simulink library "nmc"  (R2015b)
settings: Solver=ode45  SolverMode=SingleTasking  StartTime=0.0  StopTime=10.0  RelTol=1e-3
undefined symbols (not defined in the file): c, c_jointstop, CtrlPar_FP_List, CtrlPar_FP_R_List, CtrlPar_LL_List, CtrlPar_St_List, CtrlPar_St_R_List, CtrlPar_Sw_List, CtrlPar_Sw_R_List, CtrlPar_theta0_List, CtrlPar_Tr_List, CtrlPar_Tr_R_List, CtrlPar_VelocityFile_List, D1G_HAT, eref, FmaxBFSH, FmaxGAS, FmaxGLU, FmaxHAB, FmaxHAD, FmaxHAM, FmaxHFL, FmaxRF, FmaxSOL, FmaxTA, FmaxVAS, init_a_tgt, init_a_tgtR, K, leg_l, LongDelay, LongLoopDelay, loptBFSH, loptGAS, loptGLU, loptHAB, loptHAD, loptHAM, loptHFL, loptRF, loptSOL, loptTA, loptVAS, lslackBFSH, lslackGAS, lslackGLU, lslackHAB, lslackHAD, lslackHAM, lslackHFL, lslackRF, lslackSOL, lslackTA, lslackVAS, magnitude, maxLoad_control_List, MidDelay, N, phi12_LowLimit, phi12_UpLimit ... (+96)
libraries: nmc x63, simulink_extras x30, simulink x15, LopesDevelopmentLibrary x3
(part 2 of 10)

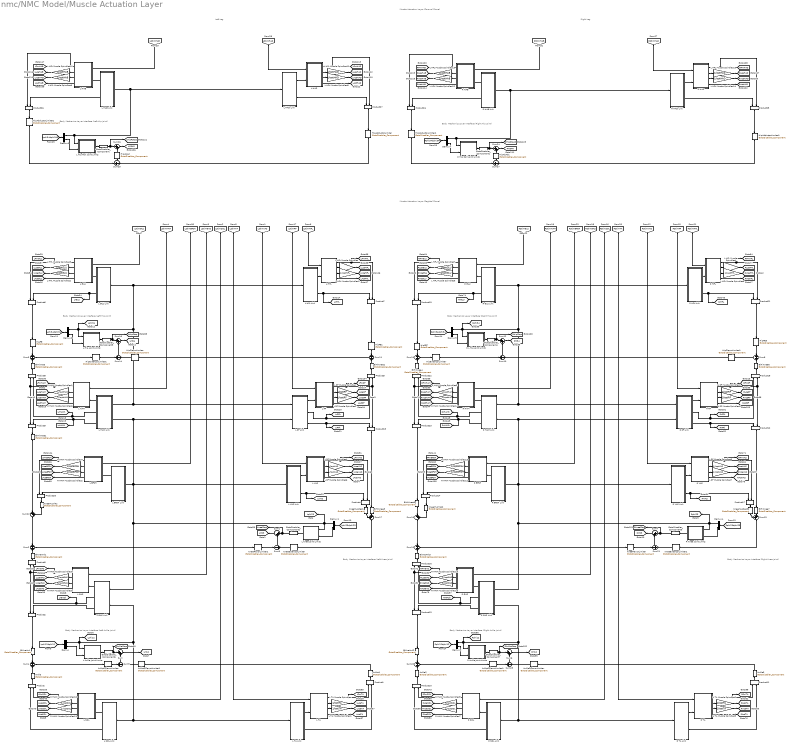
== system nmc/NMC Model/Muscle Actuation Layer ==
  note: Muscle Actuation Layer
      | (Sagittal Plane)
  note: Body Mechanics Layer
      | Interface (Left Hip Joint)
  note: Body Mechanics Layer
      | Interface (Left Knee Joint)
  note: Body Mechanics Layer
      | Interface (Left Ankle Joint)
  note: Body Mechanics Layer
      | Interface (Right Hip Joint)
  note: Body Mechanics Layer
      | Interface (Right Knee Joint)
  note: Body Mechanics Layer
      | Interface (Right Ankle Joint)
  note: Left Leg
  note: Body Mechanics Layer
      | Interface (Left Hip Joint)
  note: Body Mechanics Layer
      | Interface (Right Hip Joint)
  note: Right Leg
  note: Muscle Actuation Layer
      | (Coronal Plane)
  Ankle{,1..3} (4 alike) : nmc/GotoDisabler_Component  GotoTag=NMC_AnkleMuscles_Percentage
  AnkleDFlexorLimiter : nmc/GotoDisabler_Component  GotoTag=NMC_AnkleDFlexor_Percentage
  AnkleDFlexorLimiter1 : nmc/GotoDisabler_Component  GotoTag=NMC_AnkleDFlexor_Percentage
  AnklePFlexorLimiter : nmc/GotoDisabler_Component  GotoTag=NMC_AnklePFlexor_Percentage
  AnklePFlexorLimiter1 : nmc/GotoDisabler_Component  GotoTag=NMC_AnklePFlexor_Percentage
  BiHiKnee{,1..7} (8 alike) : nmc/GotoDisabler_Component  GotoTag=NMC_BiArticularMuscles_HK_Percentage
  BiKneAnk{,1..3} (4 alike) : nmc/GotoDisabler_Component  GotoTag=NMC_BiArticularMuscles_KA_Percentage
  Demux{,1..7} (8 alike) : Demux  Outputs=2
  GotoDisabler_Component{,1..7} (8 alike) : nmc/GotoDisabler_Component  GotoTag=DisableNMC_JointLimits
  HipAbAd : nmc/GotoDisabler_Component  GotoTag=NMC_HipAbAdMuscles_Percentage
  HipAbAd1 : nmc/GotoDisabler_Component  GotoTag=NMC_HipAbAdMuscles_Percentage
  HipAbductorLimiter1 : nmc/GotoDisabler_Component  GotoTag=NMC_HipAbductor_Percentage
  HipAbductorLimiter2 : nmc/GotoDisabler_Component  GotoTag=NMC_HipAbductor_Percentage
  HipAdductorLimiter : nmc/GotoDisabler_Component  GotoTag=NMC_HipAdductor_Percentage
  HipAdductorLimiter1 : nmc/GotoDisabler_Component  GotoTag=NMC_HipAdductor_Percentage
  HipExtensorLimiter : nmc/GotoDisabler_Component  GotoTag=NMC_HipExtensor_Percentage
  HipExtensorLimiter1 : nmc/GotoDisabler_Component  GotoTag=NMC_HipExtensor_Percentage
  HipFE{,1..3} (4 alike) : nmc/GotoDisabler_Component  GotoTag=NMC_HipFEMuscles_Percentage
  HipFlexorLimiter : nmc/GotoDisabler_Component  GotoTag=NMC_HipFlexor_Percentage
  HipFlexorLimiter1 : nmc/GotoDisabler_Component  GotoTag=NMC_HipFlexor_Percentage
  KneeExtensorLimiter : nmc/GotoDisabler_Component  GotoTag=NMC_KneeExtensor_Percentage
  KneeExtensorLimiter1 : nmc/GotoDisabler_Component  GotoTag=NMC_KneeExtensor_Percentage
  KneeFlexorLimiter : nmc/GotoDisabler_Component  GotoTag=NMC_KneeFlexor_Percentage
  KneeFlexorLimiter1 : nmc/GotoDisabler_Component  GotoTag=NMC_KneeFlexor_Percentage
  KneeMuscles{,1..3} (4 alike) : nmc/GotoDisabler_Component  GotoTag=NMC_KneeMuscles_Percentage
  L Ankle Joint Limits : Subsystem
  L BFSH : Subsystem
  L BFSH Link : Subsystem
  L GAS : Subsystem
  L GAS Link : Subsystem
  L GLU : Subsystem
  L GLU Link : Subsystem
  L HAB : Subsystem
  L HAB Link : Subsystem
  L HAD : Subsystem
  L HAD Link : Subsystem
  L HAM : Subsystem
  L HAM Link : Subsystem
  L HFL : Subsystem
  L HFL Muscle Spindles{,1,4..5} (4 alike) : Gain  Gain=1/loptHFL
  L HFL Muscle Spindles{9..10,12..13} (4 alike) : Gain  Gain=1/loptHAB
  L HFL Muscle Spindles{8,11,14..15} (4 alike) : Gain  Gain=1/loptHAD
  L HFL Muscle Spindles{2..3,6..7} (4 alike) : Gain  Gain=1/loptGLU
  L HFL Link : Subsystem
  L Hip Joint Limits : Subsystem
  L Hip Roll Joint Limits : Subsystem
  L Knee Joint Limits : Subsystem
  L RF : Subsystem
  L RF Muscle Spindles{,1..3} (4 alike) : Gain  Gain=1/loptRF
  L RF Muscle Spindles{4..7} (4 alike) : Gain  Gain=1/loptVAS
  L RF Link : Subsystem
  L SOL : Subsystem
  L SOL Link : Subsystem
  L TA : Subsystem
  L TA Muscle Spindles{,1..3} (4 alike) : Gain  Gain=1/loptTA
  L TA Link : Subsystem
  L VAS : Subsystem
  L VAS Link : Subsystem
  Product{,1..27} (28 alike) : Product  RndMeth=Zero
  R Ankle Joint Limits : Subsystem
  R BFSH : Subsystem
  R BFSH Link : Subsystem
  R GAS : Subsystem
  R GAS Link : Subsystem
  R GLU : Subsystem
  R GLU Link : Subsystem
  R HAB : Subsystem
  R HAB Link : Subsystem
  R HAD : Subsystem
  R HAD Link : Subsystem
  R HAM : Subsystem
  R HAM Muscle Spindles{1,3,6,14} (4 alike) : Gain  Gain=1/loptHAM
  R HAM Muscle Spindles{5,7,10..11} (4 alike) : Gain  Gain=1/loptSOL
  R HAM Muscle Spindles{2,4,12..13} (4 alike) : Gain  Gain=1/loptBFSH
  R HAM Muscle Spindles{8..9,15..16} (4 alike) : Gain  Gain=1/loptGAS
  R HAM Link : Subsystem
  R HFL : Subsystem
  R HFL Link : Subsystem
  R Hip Roll Joint Limits : Subsystem
  R Knee Joint Limits : Subsystem
  R L Hip Joint Limits : Subsystem
  R RF : Subsystem
  R RF Link : Subsystem
  R SOL : Subsystem
  R SOL Link : Subsystem
  R TA : Subsystem
  R TA Link : Subsystem
  R VAS : Subsystem
  R VAS Link : Subsystem
  Sum{,1,6..7,12,16,18,22,24,26} (10 alike) : Sum  Inputs=|++
  Sum{9..10,14,23,25,27} (6 alike) : Sum  Inputs=+-
  Sum{2..4,8,11,15,19..20} (8 alike) : Sum
  Sum13 : Sum  Inputs=++|
  Sum17 : Sum  Inputs=++|
  Sum21 : Sum  Inputs=-+
  Sum5 : Sum  Inputs=-+
  tag scope: LActBFSH=global, LActGAS=global, LActGLU=global, LActHAB=global, LActHAD=global, LActHAM=global, LActHFL=global, LActRF=global, LActSOL=global, LActTA=global, LActVAS=global, LAnkleStop=global, LFmBFSH=global, LFmGAS=global, LFmGLU=global, LFmHAB=global, LFmHAD=global, LFmHAM=global, LFmHFL=global, LFmRF=global, LFmSOL=global, LFmTA=global, LFmVAS=global, LHipRStop=global, LHipStop=global, LKneeStop=global, LLceBFSH=global, LLceGAS=global, LLceGLU=global, LLceHAB=global, LLceHAD=global, LLceHAM=global, LLceHFL=global, LLceRF=global, LLceSOL=global, LLceTA=global, LLceVAS=global, LM12=global, LM23=global, LM34=global, LM34R=global, LVceBFSH=global, LVceGAS=global, LVceGLU=global, LVceHAB=global, LVceHAD=global, LVceHAM=global, LVceHFL=global, LVceRF=global, LVceSOL=global, LVceTA=global, LVceVAS=global, Lphi12=global, Lphi23=global, Lphi34=global, LrGASk=global, LrGLU=global, LrHAMh=global, LrHAMk=global, LrHFL=global, LrRFh=global, LrRFk=global, LrVAS=global, RActBFSH=global, RActGAS=global, RActGLU=global, RActHAB=global, RActHAD=global, RActHAM=global, RActHFL=global, RActRF=global, RActSOL=global, RActTA=global, RActVAS=global, RAnkleStop=global, RFmBFSH=global, RFmGAS=global, RFmGLU=global, RFmHAB=global, RFmHAD=global, RFmHAM=global, RFmHFL=global, RFmRF=global, RFmSOL=global, RFmTA=global, RFmVAS=global, RHipStop=global, RHipStopR=global, RKneeStop=global, RLceBFSH=global, RLceGAS=global, RLceGLU=global, RLceHAB=global, RLceHAD=global, RLceHAM=global, RLceHFL=global, RLceRF=global, RLceSOL=global, RLceTA=global, RLceVAS=global, RM12=global, RM23=global, RM34=global, RM34R=global, RVceBFSH=global, RVceGAS=global, RVceGLU=global, RVceHAB=global, RVceHAD=global, RVceHAM=global, RVceHFL=global, RVceRF=global, RVceSOL=global, RVceTA=global, RVceVAS=global, Rphi12=global, Rphi23=global, Rphi34=global, RrGASk=global, RrGLU=global, RrHAMh=global, RrHAMk=global, RrHFL=global, RrRFh=global, RrRFk=global, RrVAS=global
  wires:
  Demux1/1 -> L Knee Joint Limits/1(phi [rad]), L VAS Link/1(phi23 [rad]), L RF Link/2(phi23 [rad]), L HAM Link/2(phi23 [rad]), L BFSH Link/1(phi23 [rad]), L GAS Link/1(phi23 [rad]), [Lphi23]
  L SOL/1(Fmtc) -> Product/2, [LFmSOL]
  L TA/2(Lce) -> L TA Muscle Spindles/1
  L TA/4(A) -> [LActTA]
  L GAS/1(Fmtc) -> Product2/1, Product3/1, [LFmGAS]
  Demux/1 -> L SOL Link/1(phi12 [rad]), L TA Link/1(phi12 [rad]), L GAS Link/2(phi12 [rad]), L Ankle Joint Limits/1(phi [rad]), [Lphi12]
  [LStimTA] -> L TA/1(STIM)
  [LStimSOL] -> L SOL/1(STIM)
  [LStimHAM] -> L HAM/1(STIM)
  L HAM/1(Fmtc) -> Product9/1, Product8/1, [LFmHAM]
  L HAM/2(Lce) -> R HAM Muscle Spindles1/1
  L HFL/2(Lce) -> L HFL Muscle Spindles/1
  L GLU/1(Fmtc) -> Product6/1, [LFmGLU]
  [LStimGLU] -> L GLU/1(STIM)
  Sum16/1 -> [LM34]
  Demux/2 -> L Ankle Joint Limits/2(dphi [rad/s])
  Sum9/1 -> Sum/2
  Demux1/2 -> L Knee Joint Limits/2(dphi [rad/s])
  L SOL Link/1(lmtc [m]) -> L SOL/2(lmtc [m])
  L TA Link/1(lmtc [m]) -> L TA/2(lmtc [m])
  L GAS Link/3(lever12 [m]) -> Product2/2
  L GAS Link/2(lever23 [m]) -> Product3/2, [LrGASk]
  [LStimGAS] -> L GAS/1(STIM)
  L GAS Link/1(lmtu [m]) -> L GAS/2(lmtc [m])
  L VAS Link/1(lmtu [m]) -> L VAS/2(lmtc [m])
  L HAM Link/1(lmtu [m]) -> L HAM/2(lmtc [m])
  L HAM Link/2(lever34 [m]) -> Product8/2, [LrHAMh]
  L HAM Link/3(lever23 [m]) -> Product9/2, [LrHAMk]
  Sum3/1 -> HipExtensorLimiter1/1
  Sum4/1 -> AnklePFlexorLimiter/1
  [Lphi12dphi12] -> Demux/1
  [Lphi23dphi23] -> Demux1/1
  [Lphi34dphi34] -> Demux2/1
  Demux2/1 -> L Hip Joint Limits/1(phi [rad]), L HFL Link/1(phi34 [rad]), L GLU Link/1(phi34 [rad]), L RF Link/1(phi34 [rad]), L HAM Link/1(phi34 [rad]), [Lphi34]
  L SOL Link/2(lever [m]) -> Product/1
  Product2/1 -> BiKneAnk/1
  L TA Link/2(lever [m]) -> Product1/2
  L Ankle Joint Limits/1(M_stop [Nm]) -> GotoDisabler_Component6/1
  L SOL/4(A) -> [LActSOL]
  L GAS/4(A) -> [LActGAS]
  L VAS/4(A) -> [LActVAS]
  L VAS/1(Fmtc) -> Product4/2, [LFmVAS]
  Sum1/1 -> [LM23]
  L Knee Joint Limits/1(M_stop [Nm]) -> GotoDisabler_Component2/1
  Sum5/1 -> Sum1/2
  L VAS Link/2(lever [m]) -> [LrVAS], Product4/1
  Sum2/1 -> KneeFlexorLimiter1/1
  L HAM/4(A) -> [LActHAM]
  L GLU Link/1(lmtu [m]) -> L GLU/2(lmtc [m])
  L GLU Link/2(lever [m]) -> Product6/2, [LrGLU]
  L GLU/4(A) -> [LActGLU]
  Demux2/2 -> L Hip Joint Limits/2(dphi [rad/s])
  Sum14/1 -> Sum16/2
  L HFL Link/1(lmtu [m]) -> L HFL/2(lmtc [m])
  L HFL/4(A) -> [LActHFL]
  L HFL Link/2(lever [m]) -> Product7/1, [LrHFL]
  [LStimVAS] -> L VAS/1(STIM)
  L GLU/2(Lce) -> L HFL Muscle Spindles3/1
  L GLU/3(Vce) -> L HFL Muscle Spindles2/1
  L HAM/3(Vce) -> R HAM Muscle Spindles6/1
  L GAS/3(Vce) -> R HAM Muscle Spindles9/1
  L GAS/2(Lce) -> R HAM Muscle Spindles8/1
  L SOL/2(Lce) -> R HAM Muscle Spindles10/1
  L SOL/3(Vce) -> R HAM Muscle Spindles11/1
  L TA/3(Vce) -> L TA Muscle Spindles1/1
  L VAS/3(Vce) -> L RF Muscle Spindles6/1
  L VAS/2(Lce) -> L RF Muscle Spindles4/1
  L HFL/3(Vce) -> L HFL Muscle Spindles1/1
  L RF/4(A) -> [LActRF]
  L RF/3(Vce) -> L RF Muscle Spindles2/1
  L RF/2(Lce) -> L RF Muscle Spindles/1
  L RF Link/1(lmtu [m]) -> L RF/2(lmtc [m])
  L RF Link/2(lever34 [m]) -> Product5/1, [LrRFh]
  L RF Link/3(lever23 [m]) -> Product15/1, [LrRFk]
  [LStimRF] -> L RF/1(STIM)
  Product5/1 -> BiHiKnee2/1
  Product15/1 -> BiHiKnee3/1
  Sum17/1 -> KneeExtensorLimiter/1
  [LStimBFSH] -> L BFSH/1(STIM)
  L BFSH Link/1(lmtu [m]) -> L BFSH/2(lmtc [m])
  L BFSH Link/2(lever [m]) -> Product20/2
  L BFSH/4(A) -> [LActBFSH]
  L BFSH/2(Lce) -> R HAM Muscle Spindles4/1
  L BFSH/3(Vce) -> R HAM Muscle Spindles2/1
  L HFL Muscle Spindles1/1 -> [LVceHFL]
  L HFL Muscle Spindles2/1 -> [LVceGLU]
  L HFL Muscle Spindles3/1 -> [LLceGLU]
  L RF Muscle Spindles6/1 -> [LVceVAS]
  L RF/1(Fmtc) -> Product5/2, Product15/2, [LFmRF]
  L BFSH/1(Fmtc) -> Product20/1, [LFmBFSH]
  R HAM Muscle Spindles8/1 -> [LLceGAS]
  R HAM Muscle Spindles9/1 -> [LVceGAS]
  R HAM Muscle Spindles10/1 -> [LLceSOL]
  R HAM Muscle Spindles11/1 -> [LVceSOL]
  L TA/1(Fmtc) -> Product1/1, [LFmTA]
  L TA Muscle Spindles1/1 -> [LVceTA]
  L HFL Muscle Spindles/1 -> [LLceHFL]
  R HAM Muscle Spindles1/1 -> [LLceHAM]
  R HAM Muscle Spindles6/1 -> [LVceHAM]
  L RF Muscle Spindles/1 -> [LLceRF]
  L RF Muscle Spindles2/1 -> [LVceRF]
  R HAM Muscle Spindles4/1 -> [LLceBFSH]
  R HAM Muscle Spindles2/1 -> [LVceBFSH]
  L RF Muscle Spindles4/1 -> [LLceVAS]
  L TA Muscle Spindles/1 -> [LLceTA]
  Demux4/1 -> R Knee Joint Limits/1(phi [rad]), R VAS Link/1(phi23 [rad]), R RF Link/2(phi23 [rad]), R HAM Link/2(phi23 [rad]), R BFSH Link/1(phi23 [rad]), R GAS Link/1(phi23 [rad]), [Rphi23]
  R SOL/1(Fmtc) -> Product10/2, [RFmSOL]
  R TA/2(Lce) -> L TA Muscle Spindles2/1
  R TA/4(A) -> [RActTA]
  R GAS/1(Fmtc) -> Product13/1, Product16/1, [RFmGAS]
  Demux3/1 -> R SOL Link/1(phi12 [rad]), R TA Link/1(phi12 [rad]), R GAS Link/2(phi12 [rad]), R Ankle Joint Limits/1(phi [rad]), [Rphi12]
  [RStimTA] -> R TA/1(STIM)
  [RStimSOL] -> R SOL/1(STIM)
  [RStimHAM] -> R HAM/1(STIM)
  R HAM/1(Fmtc) -> Product23/1, Product22/1, [RFmHAM]
  R HAM/2(Lce) -> R HAM Muscle Spindles3/1
  R HFL/1(Fmtc) -> Product21/2, [RFmHFL]
  R HFL/2(Lce) -> L HFL Muscle Spindles4/1
  [RStimHFL] -> R HFL/1(STIM)
  R GLU/1(Fmtc) -> Product19/1, [RFmGLU]
  [RStimGLU] -> R GLU/1(STIM)
  Sum12/1 -> [RM34]
  Demux3/2 -> R Ankle Joint Limits/2(dphi [rad/s])
  Sum23/1 -> Sum6/2
  Demux4/2 -> R Knee Joint Limits/2(dphi [rad/s])
  R SOL Link/1(lmtc [m]) -> R SOL/2(lmtc [m])
  R TA Link/1(lmtc [m]) -> R TA/2(lmtc [m])
  R GAS Link/3(lever12 [m]) -> Product13/2
  R GAS Link/2(lever23 [m]) -> Product16/2, [RrGASk]
  [RStimGAS] -> R GAS/1(STIM)
  R GAS Link/1(lmtu [m]) -> R GAS/2(lmtc [m])
  R VAS Link/1(lmtu [m]) -> R VAS/2(lmtc [m])
  R HAM Link/1(lmtu [m]) -> R HAM/2(lmtc [m])
  R HAM Link/2(lever34 [m]) -> Product22/2, [RrHAMh]
  R HAM Link/3(lever23 [m]) -> Product23/2, [RrHAMk]
  Sum19/1 -> HipExtensorLimiter/1
  Sum20/1 -> AnklePFlexorLimiter1/1
  [Rphi12dphi12] -> Demux3/1
  [Rphi23dphi23] -> Demux4/1
  [Rphi34dphi34] -> Demux5/1
  Demux5/1 -> R L Hip Joint Limits/1(phi [rad]), R HFL Link/1(phi34 [rad]), R GLU Link/1(phi34 [rad]), R RF Link/1(phi34 [rad]), R HAM Link/1(phi34 [rad]), [Rphi34]
  R SOL Link/2(lever [m]) -> Product10/1
  Product13/1 -> BiKneAnk2/1
  R TA Link/2(lever [m]) -> Product11/2
  Sum6/1 -> [RM12]
  R SOL/4(A) -> [RActSOL]
  R GAS/4(A) -> [RActGAS]
  R VAS/4(A) -> [RActVAS]
  R VAS/1(Fmtc) -> Product17/2, [RFmVAS]
  Sum7/1 -> [RM23]
  R Knee Joint Limits/1(M_stop [Nm]) -> GotoDisabler_Component3/1
  Sum21/1 -> Sum7/2
  R VAS Link/2(lever [m]) -> [RrVAS], Product17/1
  Sum15/1 -> KneeFlexorLimiter/1
  R HAM/4(A) -> [RActHAM]
  Product22/1 -> BiHiKnee4/1
  R GLU Link/1(lmtu [m]) -> R GLU/2(lmtc [m])
  R GLU Link/2(lever [m]) -> Product19/2, [RrGLU]
  R GLU/4(A) -> [RActGLU]
  Demux5/2 -> R L Hip Joint Limits/2(dphi [rad/s])
  Sum10/1 -> Sum12/2
  R HFL Link/1(lmtu [m]) -> R HFL/2(lmtc [m])
  R HFL/4(A) -> [RActHFL]
  R HFL Link/2(lever [m]) -> Product21/1, [RrHFL]
  [RStimVAS] -> R VAS/1(STIM)
  R GLU/2(Lce) -> L HFL Muscle Spindles7/1
  R GLU/3(Vce) -> L HFL Muscle Spindles6/1
  R HAM/3(Vce) -> R HAM Muscle Spindles14/1
  R GAS/3(Vce) -> R HAM Muscle Spindles16/1
  R GAS/2(Lce) -> R HAM Muscle Spindles15/1
  R SOL/2(Lce) -> R HAM Muscle Spindles5/1
  R SOL/3(Vce) -> R HAM Muscle Spindles7/1
  R TA/3(Vce) -> L TA Muscle Spindles3/1
  R VAS/3(Vce) -> L RF Muscle Spindles7/1
  R VAS/2(Lce) -> L RF Muscle Spindles5/1
  R HFL/3(Vce) -> L HFL Muscle Spindles5/1
  R RF/4(A) -> [RActRF]
  R RF/3(Vce) -> L RF Muscle Spindles3/1
  R RF/2(Lce) -> L RF Muscle Spindles1/1
  R RF Link/1(lmtu [m]) -> R RF/2(lmtc [m])
  R RF Link/2(lever34 [m]) -> Product18/1, [RrRFh]
  R RF Link/3(lever23 [m]) -> Product12/1, [RrRFk]
  [RStimRF] -> R RF/1(STIM)
  Sum8/1 -> HipFlexorLimiter1/1
  Product18/1 -> BiHiKnee6/1
  Product12/1 -> BiHiKnee7/1
  Sum13/1 -> KneeExtensorLimiter1/1
  [RStimBFSH] -> R BFSH/1(STIM)
  R BFSH Link/1(lmtu [m]) -> R BFSH/2(lmtc [m])
  R BFSH Link/2(lever [m]) -> Product14/2
  R BFSH/4(A) -> [RActBFSH]
  R BFSH/2(Lce) -> R HAM Muscle Spindles13/1
  R BFSH/3(Vce) -> R HAM Muscle Spindles12/1
  Sum18/1 -> Sum15/1
  Product23/1 -> BiHiKnee5/1
  L HFL Muscle Spindles5/1 -> [RVceHFL]
  L HFL Muscle Spindles6/1 -> [RVceGLU]
  L HFL Muscle Spindles7/1 -> [RLceGLU]
  L RF Muscle Spindles7/1 -> [RVceVAS]
  R RF/1(Fmtc) -> Product18/2, Product12/2, [RFmRF]
  R BFSH/1(Fmtc) -> Product14/1, [RFmBFSH]
  R HAM Muscle Spindles15/1 -> [RLceGAS]
  R HAM Muscle Spindles16/1 -> [RVceGAS]
  R HAM Muscle Spindles5/1 -> [RLceSOL]
  R HAM Muscle Spindles7/1 -> [RVceSOL]
  R TA/1(Fmtc) -> Product11/1, [RFmTA]
  L TA Muscle Spindles3/1 -> [RVceTA]
  L HFL Muscle Spindles4/1 -> [RLceHFL]
  R HAM Muscle Spindles3/1 -> [RLceHAM]
  R HAM Muscle Spindles14/1 -> [RVceHAM]
  L RF Muscle Spindles1/1 -> [RLceRF]
  L RF Muscle Spindles3/1 -> [RVceRF]
  R HAM Muscle Spindles13/1 -> [RLceBFSH]
  R HAM Muscle Spindles12/1 -> [RVceBFSH]
  L RF Muscle Spindles5/1 -> [RLceVAS]
  L TA Muscle Spindles2/1 -> [RLceTA]
  Sum11/1 -> HipFlexorLimiter/1
  [LStimHAD] -> L HAD/1(STIM)
  [LStimHAB] -> L HAB/1(STIM)
  Sum26/1 -> [LM34R]
  [Lphi34dphi34R] -> Demux6/1
  Demux6/1 -> L HAB Link/1(phi34R [rad]), L HAD Link/1(phi34R [rad]), L Hip Roll Joint Limits/1(phi [rad])
  Product26/1 -> HipAbductorLimiter2/1
  L HAB Link/1(lmtu [m]) -> L HAB/2(lmtc [m])
  L HAB Link/2(lever [m]) -> Product26/2
  Demux6/2 -> L Hip Roll Joint Limits/2(dphi [rad/s])
  L Hip Roll Joint Limits/1(M_stop [Nm]) -> GotoDisabler_Component/1
  Product27/1 -> HipAdductorLimiter/1
  L HAD Link/1(lmtu [m]) -> L HAD/2(lmtc [m])
  L HAD Link/2(lever [m]) -> Product27/1
  [RStimHAD] -> R HAD/1(STIM)
  Sum24/1 -> [RM34R]
  [Rphi34dphi34R] -> Demux7/1
  Demux7/1 -> R HAD Link/1(phi34R [rad]), R HAB Link/1(phi34R [rad]), R Hip Roll Joint Limits/1(phi [rad])
  Product24/1 -> HipAbductorLimiter1/1
  R HAB Link/1(lmtu [m]) -> R HAB/2(lmtc [m])
  R HAB Link/2(lever [m]) -> Product24/2
  Demux7/2 -> R Hip Roll Joint Limits/2(dphi [rad/s])
  R Hip Roll Joint Limits/1(M_stop [Nm]) -> GotoDisabler_Component1/1
  Product25/1 -> HipAdductorLimiter1/1
  R HAD Link/1(lmtu [m]) -> R HAD/2(lmtc [m])
  R HAD Link/2(lever [m]) -> Product25/1
  [RStimHAB] -> R HAB/1(STIM)
  L HAB/4(A) -> [LActHAB]
  L HAB/2(Lce) -> L HFL Muscle Spindles10/1
  L HAB/3(Vce) -> L HFL Muscle Spindles9/1
  L HFL Muscle Spindles9/1 -> [LVceHAB]
  L HFL Muscle Spindles10/1 -> [LLceHAB]
  L HAB/1(Fmtc) -> Product26/1, [LFmHAB]
  L HFL Muscle Spindles8/1 -> [LVceHAD]
  L HFL Muscle Spindles11/1 -> [LLceHAD]
  L HAD/2(Lce) -> L HFL Muscle Spindles11/1
  L HAD/3(Vce) -> L HFL Muscle Spindles8/1
  L HAD/4(A) -> [LActHAD]
  L HAD/1(Fmtc) -> [LFmHAD], Product27/2
  R HAB/4(A) -> [RActHAB]
  R HAB/2(Lce) -> L HFL Muscle Spindles13/1
  R HAB/3(Vce) -> L HFL Muscle Spindles12/1
  L HFL Muscle Spindles12/1 -> [RVceHAB]
  L HFL Muscle Spindles13/1 -> [RLceHAB]
  R HAB/1(Fmtc) -> [RFmHAB], Product24/1
  L HFL Muscle Spindles14/1 -> [RVceHAD]
  L HFL Muscle Spindles15/1 -> [RLceHAD]
  R HAD/2(Lce) -> L HFL Muscle Spindles15/1
  R HAD/3(Vce) -> L HFL Muscle Spindles14/1
  R HAD/4(A) -> [RActHAD]
  R HAD/1(Fmtc) -> [RFmHAD], Product25/2
  Sum/1 -> [LM12]
  GotoDisabler_Component7/1 -> Sum6/1, [RAnkleStop]
  GotoDisabler_Component6/1 -> Sum/1, [LAnkleStop]
  GotoDisabler_Component3/1 -> Sum7/1, [RKneeStop]
  GotoDisabler_Component2/1 -> Sum1/1, [LKneeStop]
  GotoDisabler_Component/1 -> Sum26/1, [LHipRStop]
  GotoDisabler_Component1/1 -> Sum24/1, [RHipStopR]
  R L Hip Joint Limits/1(M_stop [Nm]) -> GotoDisabler_Component4/1
  GotoDisabler_Component4/1 -> [RHipStop], Sum12/1
  L Hip Joint Limits/1(M_stop [Nm]) -> GotoDisabler_Component5/1
  GotoDisabler_Component5/1 -> Sum16/1, [LHipStop]
  R Ankle Joint Limits/1(M_stop [Nm]) -> GotoDisabler_Component7/1
  Product4/1 -> KneeMuscles1/1
  Product17/1 -> KneeMuscles3/1
  Product14/1 -> KneeMuscles2/1
  Product20/1 -> KneeMuscles/1
  Product21/1 -> HipFE3/1
  Product19/1 -> HipFE2/1
  Product6/1 -> HipFE/1
  Product/1 -> Ankle/1
  Product10/1 -> Ankle2/1
  Product11/1 -> Ankle3/1
  Product1/1 -> Ankle1/1
  HipAbductorLimiter2/1 -> Sum25/1
  HipAbductorLimiter1/1 -> Sum27/1
  HipAdductorLimiter/1 -> Sum25/2
  HipAdductorLimiter1/1 -> Sum27/2
  Product9/1 -> BiHiKnee1/1
  KneeFlexorLimiter1/1 -> Sum5/1
  KneeExtensorLimiter/1 -> Sum5/2
  KneeFlexorLimiter/1 -> Sum21/1
  KneeExtensorLimiter1/1 -> Sum21/2
  AnklePFlexorLimiter1/1 -> Sum23/1
  AnklePFlexorLimiter/1 -> Sum9/1
  HipExtensorLimiter1/1 -> Sum14/1
  HipFlexorLimiter/1 -> Sum14/2
  HipExtensorLimiter/1 -> Sum10/1
  HipFlexorLimiter1/1 -> Sum10/2
  AnkleDFlexorLimiter1/1 -> Sum9/2
  AnkleDFlexorLimiter/1 -> Sum23/2
  Sum25/1 -> HipAbAd/1
  HipAbAd/1 -> Sum26/2
  Sum27/1 -> HipAbAd1/1
  HipAbAd1/1 -> Sum24/2
  HipFE/1 -> Sum3/1
  HipFE1/1 -> Sum11/1
  HipFE2/1 -> Sum19/1
  HipFE3/1 -> Sum8/1
  BiHiKnee/1 -> Sum3/2
  Product8/1 -> BiHiKnee/1
  BiHiKnee1/1 -> Sum22/1
  BiHiKnee2/1 -> Sum11/2
  BiHiKnee3/1 -> Sum17/2
  BiHiKnee4/1 -> Sum19/2
  BiHiKnee5/1 -> Sum18/1
  BiHiKnee6/1 -> Sum8/2
  BiHiKnee7/1 -> Sum13/2
  Sum22/1 -> Sum2/1
  KneeMuscles/1 -> Sum22/2
  KneeMuscles1/1 -> Sum17/1
  KneeMuscles2/1 -> Sum18/2
  KneeMuscles3/1 -> Sum13/1
  BiKneAnk/1 -> Sum4/1
  Product3/1 -> BiKneAnk1/1
  BiKneAnk1/1 -> Sum2/2
  BiKneAnk2/1 -> Sum20/1
  Product16/1 -> BiKneAnk3/1
  BiKneAnk3/1 -> Sum15/2
  Ankle/1 -> Sum4/2
  Ankle1/1 -> AnkleDFlexorLimiter1/1
  Ankle2/1 -> Sum20/2
  Ankle3/1 -> AnkleDFlexorLimiter/1
  Product7/1 -> HipFE1/1
  [LStimHFL] -> L HFL/1(STIM)
  L HFL/1(Fmtc) -> Product7/2, [LFmHFL]

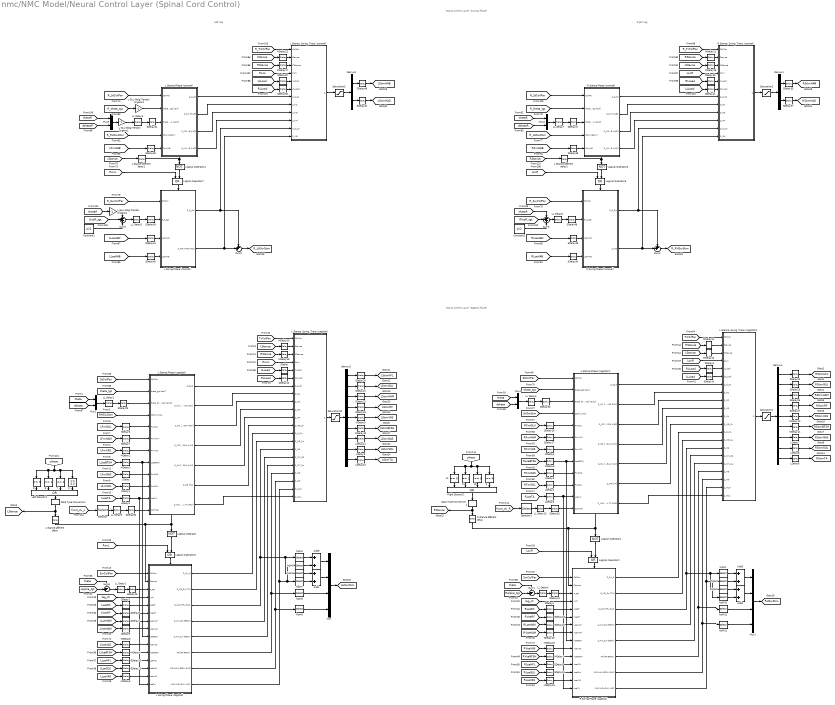
== system nmc/NMC Model/Neural Control Layer (Spinal Cord Control) ==
  note: Left Leg
  note: Right Leg
  note: Neural Control Layer
      | (Coronal Plane)
  note: Neural Control Layer
      | (Sagittal Plane)
  " 2" : simulink/Logic and Bit Operations/Compare To Constant  relop===  const=3.0  OutDataTypeStr=boolean
  " 3" : simulink/Logic and Bit Operations/Compare To Constant  relop===  const=4  OutDataTypeStr=boolean
  10 : simulink/Logic and Bit Operations/Compare To Constant  relop===  const=3  OutDataTypeStr=boolean
  11 : simulink/Logic and Bit Operations/Compare To Constant  relop===  const=1  OutDataTypeStr=boolean
  12 : simulink/Logic and Bit Operations/Compare To Constant  relop===  const=0  OutDataTypeStr=boolean
  7 : simulink/Logic and Bit Operations/Compare To Constant  relop===  const=2  OutDataTypeStr=boolean
  8 : simulink/Logic and Bit Operations/Compare To Constant  relop===  const=1  OutDataTypeStr=boolean
  9 : simulink/Logic and Bit Operations/Compare To Constant  relop===  const=0  OutDataTypeStr=boolean
  Add{1..3,9} (4 alike) : Sum  Inputs=2
  Constant1 : Constant  Value=pi/2
  Constant2 : Constant  Value=pi/2
  Data Type Conversion : DataTypeConversion
  Data Type Conversion1 : DataTypeConversion
  Demux1 : Demux  Outputs=2
  Demux2 : Demux  Outputs=2
  Demux3 : Demux  Outputs=9
  Demux4 : Demux  Outputs=9
  L GLU Golgi Tendon Organs1 : Gain  Gain=-1
  L GLU Golgi Tendon Organs2 : Gain  Gain=-1
  L GLU Golgi Tendon Organs3 : Gain  Gain=-1
  L Stance afferent delay : TransportDelay  DelayTime=MidDelay
  L Stance afferent delay1 : TransportDelay  DelayTime=MidDelay
  L Stance afferent delay2 : TransportDelay  DelayTime=MidDelay
  L Stance Phase (coronal) : Subsystem  TreatAsAtomicUnit=on
  L Stance Phase (sagittal) : Subsystem  TreatAsAtomicUnit=on
  L Stance Phase (sagittal)1 : Subsystem  TreatAsAtomicUnit=on
  "L Stance, Swing, Trans (coronal)" : Subsystem  TreatAsAtomicUnit=on
  "L Stance, Swing, Trans (sagittal)" : Subsystem
  "L Stance, Swing, Trans (sagittal)1" : Subsystem
  L Swing Phase (coronal) : Subsystem  TreatAsAtomicUnit=on
  L Swing Phase (sagittal) : Subsystem  TreatAsAtomicUnit=on
  LDelay{,1,3..4} (4 alike) : TransportDelay  DelayTime=LongDelay
  LDelay10 : TransportDelay  DelayTime=LongDelay  InitialOutput=St_PreSTA
  LDelay11 : TransportDelay  DelayTime=LongDelay  InitialOutput=St_PreSGAS
  LDelay2 : TransportDelay  DelayTime=LongDelay  InitialOutput=1
  LDelay5 : TransportDelay  DelayTime=LongDelay  InitialOutput=1
  LDelay6 : TransportDelay  DelayTime=LongDelay  InitialOutput=Sw_PreSTA
  LDelay7 : TransportDelay  DelayTime=LongDelay  InitialOutput=Sw_PreSGAS
  LDelay8 : TransportDelay  DelayTime=LongDelay  InitialOutput=Sw_PreSSOL
  LDelay9 : TransportDelay  DelayTime=LongDelay  InitialOutput=St_PreSSOL
  LL Delay1 : TransportDelay  DelayTime=LongLoopDelay/2  InitialOutput=init_a_tgt
  LL Delay{2..3,6..7,9..10} (6 alike) : TransportDelay  DelayTime=LongLoopDelay/2
  LL Delay4 : TransportDelay  DelayTime=LongLoopDelay/2  InitialOutput=init_a_tgt
  LL Delay5 : TransportDelay  DelayTime=LongLoopDelay/2  InitialOutput=init_a_tgtR
  LL Delay8 : TransportDelay  DelayTime=LongLoopDelay/2  InitialOutput=init_a_tgtR
  Left Stance?2 : Logic  Operator=OR  Inputs=4  AllPortsSameDT=off
  Logical Operator{,1,4..5} (4 alike) : Logic  Operator=NOT  AllPortsSameDT=off  OutDataTypeStr=boolean
  Logical Operator{2..3,6..7} (4 alike) : Logic  Operator=OR  AllPortsSameDT=off  OutDataTypeStr=boolean
  MDelay{1..2,4,7..8,13..14,16..22} (14 alike) : TransportDelay  DelayTime=MidDelay
  MDelay10 : TransportDelay  DelayTime=MidDelay  InitialOutput=St_PreSBFSH
  MDelay11 : TransportDelay  DelayTime=MidDelay  InitialOutput=Sw_PreSBFSH
  MDelay12 : TransportDelay  DelayTime=MidDelay  InitialOutput=Sw_PreSVAS
  MDelay{3,5..6,15} (4 alike) : TransportDelay  DelayTime=MidDelay  InitialOutput=1
  MDelay9 : TransportDelay  DelayTime=MidDelay  InitialOutput=St_PreSVAS
  Mux : Mux
  Mux1 : Mux
  Mux{2..5} (4 alike) : Mux  Inputs=2
  R Stance afferent delay : TransportDelay  DelayTime=MidDelay
  R Stance Phase (coronal) : Subsystem  TreatAsAtomicUnit=on
  "R Stance, Swing, Trans (coronal)" : Subsystem  TreatAsAtomicUnit=on
  R Swing Phase (coronal) : Subsystem  TreatAsAtomicUnit=on
  R Swing Phase (sagittal) : Subsystem  TreatAsAtomicUnit=on
  Right Stance?1 : Logic  Operator=OR  Inputs=4  AllPortsSameDT=off
  SDelay{,3,6..9,12,14,16..19,29..30,32..33,36,38..39,41..42,47,50..51} (24 alike) : TransportDelay  DelayTime=ShortDelay
  SDelay{1..2,4..5,10..11,13,15,34,44..45,49} (12 alike) : TransportDelay  DelayTime=ShortDelay  InitialOutput=1
  SDelay20 : TransportDelay  DelayTime=ShortDelay  InitialOutput=St_PreSHFL
  SDelay21 : TransportDelay  DelayTime=ShortDelay  InitialOutput=St_PreSGLU
  SDelay22 : TransportDelay  DelayTime=ShortDelay  InitialOutput=St_PreSHAM
  SDelay23 : TransportDelay  DelayTime=ShortDelay  InitialOutput=St_PreSRF
  SDelay24 : TransportDelay  DelayTime=ShortDelay  InitialOutput=Sw_PreSHFL
  SDelay25 : TransportDelay  DelayTime=ShortDelay  InitialOutput=Sw_PreSGLU
  SDelay26 : TransportDelay  DelayTime=ShortDelay  InitialOutput=Sw_PreSHAM
  SDelay27 : TransportDelay  DelayTime=ShortDelay  InitialOutput=Sw_PreSRF
  SDelay28 : TransportDelay  DelayTime=ShortDelay  InitialOutput=init_a_tgt
  SDelay31 : TransportDelay  DelayTime=ShortDelay  InitialOutput=init_a_tgt
  SDelay35 : TransportDelay  DelayTime=ShortDelay  InitialOutput=Sw_PreS_HAB
  SDelay37 : TransportDelay  DelayTime=ShortDelay  InitialOutput=Sw_PreS_HAD
  SDelay40 : TransportDelay  DelayTime=ShortDelay  InitialOutput=St_PreS_HAD
  SDelay43 : TransportDelay  DelayTime=ShortDelay  InitialOutput=init_a_tgtR
  SDelay46 : TransportDelay  DelayTime=ShortDelay  InitialOutput=St_PreS_HAB
  SDelay48 : TransportDelay  DelayTime=ShortDelay  InitialOutput=init_a_tgtR
  Saturation{1..3,10} (4 alike) : Saturate  UpperLimit=1  LowerLimit=0.01  ZeroCross=off
  Selector : Selector  InputPortWidth=2  IndexOptions=Index vector (dialog)  Indices=[2]  OutputSizes=1
  Selector1 : Selector  InputPortWidth=2  IndexOptions=Index vector (dialog)  Indices=[2]  OutputSizes=1
  Sum1 : Sum  Inputs=-+|
  Sum2 : Sum  Inputs=++|
  Sum3 : Sum  Inputs=--+
  Sum4 : Sum  Inputs=++|
  Sum5 : Sum  Inputs=--+
  Sum6 : Sum  Inputs=-+|
  hipM{1,4,9,12} (4 alike) : Selector  InputPortWidth=2  IndexOptions=Index vector (dialog)  Indices=1  OutputSizes=1
  hipM10 : Selector  InputPortWidth=3  IndexOptions=Index vector (dialog)  Indices=2  OutputSizes=1
  hipM{2,5,8,11} (4 alike) : Selector  InputPortWidth=3  IndexOptions=Index vector (dialog)  Indices=1  OutputSizes=1
  hipM3 : Selector  InputPortWidth=2  IndexOptions=Index vector (dialog)  Indices=2  OutputSizes=1
  hipM6 : Selector  InputPortWidth=2  IndexOptions=Index vector (dialog)  Indices=2  OutputSizes=1
  hipM7 : Selector  InputPortWidth=3  IndexOptions=Index vector (dialog)  Indices=2  OutputSizes=1
  tag scope: LHSwStim=global, LStance=global, LStimBFSH=global, LStimGAS=global, LStimGLU=global, LStimHAB=global, LStimHAD=global, LStimHAM=global, LStimHFL=global, LStimRF=global, LStimSOL=global, LStimTA=global, LStimVAS=global, RHSwStim=global, RStance=global, RStimBFSH=global, RStimGAS=global, RStimGLU=global, RStimHAB=global, RStimHAD=global, RStimHAM=global, RStimHFL=global, RStimRF=global, RStimSOL=global, RStimTA=global, RStimVAS=global, R_LHSwStim=global, R_RHSwStim=global
  wires:
  SDelay51/1 -> L Stance Phase (sagittal)1/12(COMVel)
  LL Delay10/1 -> SDelay51/1
  SDelay50/1 -> L Stance Phase (sagittal)/12(COMVel)
  LL Delay9/1 -> SDelay50/1
  Selector1/1 -> LL Delay10/1
  [front_dv_R] -> Selector1/1
  Selector/1 -> LL Delay9/1
  L Stance Phase (sagittal)1/7(S_M11 [SOL TA GAS]) -> "L Stance, Swing, Trans (sagittal)1"/21(S_M11)
  [front_dv_L] -> Selector/1
  L Stance Phase (sagittal)/7(S_M11 [SOL TA GAS]) -> "L Stance, Swing, Trans (sagittal)"/21(S_M11)
  SDelay37/1 -> [RStimHAD]
  SDelay35/1 -> [RStimHAB]
  SDelay39/1 -> L Stance Phase (coronal)/5(FmHAB)
  [LFmHAB] -> SDelay39/1
  L Stance Phase (coronal)/2(S_M1 [HAB]) -> "L Stance, Swing, Trans (coronal)"/8(S_M1)
  [dthetaR] -> Mux5/2
  [thetaR] -> Mux5/1
  L GLU Golgi Tendon Organs2/1 -> Sum3/1
  [thetaR] -> L GLU Golgi Tendon Organs2/1
  [LhipR_tgt] -> Sum3/2
  "L Stance, Swing, Trans (coronal)"/1(S) -> Saturation3/1
  SDelay40/1 -> [LStimHAD]
  SDelay46/1 -> [LStimHAB]
  MDelay17/1 -> "L Stance, Swing, Trans (coronal)"/3(CStance)
  MDelay22/1 -> "L Stance, Swing, Trans (coronal)"/2(Stance)
  SDelay45/1 -> L Swing Phase (coronal)/4(LceHAB)
  SDelay44/1 -> L Swing Phase (coronal)/3(LceHAD)
  Sum3/1 -> LL Delay5/1
  SDelay43/1 -> L Swing Phase (coronal)/2(R_a_tgt)
  LL Delay5/1 -> SDelay43/1
  L GLU Golgi Tendon Organs1/1 -> LL Delay6/1
  SDelay42/1 -> L Stance Phase (coronal)/3(theta dtheta [rad rad/s])
  LL Delay6/1 -> SDelay42/1
  Constant1/1 -> Sum3/3
  [LLceHAB] -> SDelay45/1
  [LLceHAD] -> SDelay44/1
  L Swing Phase (coronal)/1(S_0_Sw) -> Sum2/1, "L Stance, Swing, Trans (coronal)"/11(S_0_Sw)
  L Stance Phase (coronal)/4(S_M4 [HAB HAD]) -> "L Stance, Swing, Trans (coronal)"/10(S_M4)
  L Stance Phase (coronal)/3(S_M3 [HAB HAD]) -> "L Stance, Swing, Trans (coronal)"/9(S_M3)
  L Stance Phase (coronal)/1(S_0_St) -> "L Stance, Swing, Trans (coronal)"/7(S_0_St)
  SDelay32/1 -> "L Stance, Swing, Trans (coronal)"/5(ILLoad)
  Sum2/1 -> [R_LHSwStim]
  L Swing Phase (coronal)/2(S_M6 [HAB HAD]) -> "L Stance, Swing, Trans (coronal)"/12(S_M6), Sum2/2
  Mux5/1 -> L GLU Golgi Tendon Organs1/1
  [R_theta_tgt] -> L GLU Golgi Tendon Organs3/1
  [LLLoad] -> SDelay32/1
  Demux2/1 -> SDelay46/1
  Demux2/2 -> SDelay40/1
  Saturation3/1 -> Demux2/1
  SDelay36/1 -> "L Stance, Swing, Trans (coronal)"/6(CLLoad)
  [RLLoad] -> SDelay36/1
  [RStance] -> MDelay17/1
  [LStance] -> MDelay22/1
  [RonL] -> "L Stance, Swing, Trans (coronal)"/4(ConI)
  [R_TrCtrlPar] -> "L Stance, Swing, Trans (coronal)"/1(CtrlPar)
  [R_SwCtrlPar] -> L Swing Phase (coronal)/1(CtrlPar)
  [R_RHSwStim] -> L Stance Phase (coronal)/4(CSwingStim)
  [R_StCtrlPar] -> L Stance Phase (coronal)/1(CtrlPar)
  L GLU Golgi Tendon Organs3/1 -> L Stance Phase (coronal)/2(theta_tgt [rad])
  L Stance afferent delay1/1 -> L Stance Phase (coronal)/Enable, Logical Operator4/1
  [LStance] -> L Stance afferent delay1/1
  [RonL] -> Logical Operator7/1
  Logical Operator7/1 -> L Swing Phase (coronal)/Enable
  Logical Operator4/1 -> Logical Operator7/2
  SDelay38/1 -> R Stance Phase (coronal)/5(FmHAB)
  [RFmHAB] -> SDelay38/1
  R Stance Phase (coronal)/2(S_M1 [HAB]) -> "R Stance, Swing, Trans (coronal)"/8(S_M1)
  [dthetaR] -> Mux3/2
  [thetaR] -> Mux3/1
  "R Stance, Swing, Trans (coronal)"/1(S) -> Saturation2/1
  MDelay18/1 -> "R Stance, Swing, Trans (coronal)"/3(CStance)
  [LStance] -> MDelay18/1
  [RStance] -> MDelay21/1
  MDelay21/1 -> "R Stance, Swing, Trans (coronal)"/2(Stance)
  SDelay34/1 -> R Swing Phase (coronal)/4(LceHAB)
  SDelay49/1 -> R Swing Phase (coronal)/3(LceHAD)
  Sum5/1 -> LL Delay8/1
  SDelay48/1 -> R Swing Phase (coronal)/2(R_a_tgt)
  LL Delay8/1 -> SDelay48/1
  Mux3/1 -> LL Delay7/1
  SDelay47/1 -> R Stance Phase (coronal)/3(theta dtheta [rad rad/s])
  LL Delay7/1 -> SDelay47/1
  [thetaR] -> Sum5/1
  Constant2/1 -> Sum5/3
  [RhipR_tgt] -> Sum5/2
  [RLceHAB] -> SDelay34/1
  [RLceHAD] -> SDelay49/1
  R Swing Phase (coronal)/1(S_0_Sw) -> "R Stance, Swing, Trans (coronal)"/11(S_0_Sw), Sum4/1
  R Stance Phase (coronal)/4(S_M4 [HAB HAD]) -> "R Stance, Swing, Trans (coronal)"/10(S_M4)
  R Stance Phase (coronal)/3(S_M3 [HAB HAD]) -> "R Stance, Swing, Trans (coronal)"/9(S_M3)
  R Stance Phase (coronal)/1(S_0_St) -> "R Stance, Swing, Trans (coronal)"/7(S_0_St)
  SDelay33/1 -> "R Stance, Swing, Trans (coronal)"/5(ILLoad)
  Sum4/1 -> [R_RHSwStim]
  R Swing Phase (coronal)/2(S_M6) -> "R Stance, Swing, Trans (coronal)"/12(S_M6), Sum4/2
  [R_theta_tgt] -> R Stance Phase (coronal)/2(theta_tgt [rad])
  [RLLoad] -> SDelay33/1
  Demux1/1 -> SDelay35/1
  Demux1/2 -> SDelay37/1
  Saturation2/1 -> Demux1/1
  SDelay41/1 -> "R Stance, Swing, Trans (coronal)"/6(CLLoad)
  [LLLoad] -> SDelay41/1
  [LonR] -> "R Stance, Swing, Trans (coronal)"/4(ConI)
  [R_TrCtrlPar] -> "R Stance, Swing, Trans (coronal)"/1(CtrlPar)
  [R_SwCtrlPar] -> R Swing Phase (coronal)/1(CtrlPar)
  [R_LHSwStim] -> R Stance Phase (coronal)/4(CSwingStim)
  [R_StCtrlPar] -> R Stance Phase (coronal)/1(CtrlPar)
  L Stance afferent delay2/1 -> R Stance Phase (coronal)/Enable, Logical Operator5/1
  [RStance] -> L Stance afferent delay2/1
  [LonR] -> Logical Operator6/1
  Logical Operator6/1 -> R Swing Phase (coronal)/Enable
  Logical Operator5/1 -> Logical Operator6/2
  MDelay16/1 -> R Swing Phase (sagittal)/10(VceVAS)
  [RVceVAS] -> MDelay16/1
  MDelay8/1 -> L Swing Phase (sagittal)/10(VceVAS)
  [LVceVAS] -> MDelay8/1
  SDelay31/1 -> R Swing Phase (sagittal)/3(a_tgt)
  Sum1/1 -> LL Delay4/1
  LL Delay4/1 -> SDelay31/1
  hipM11/1 -> Mux1/4
  hipM12/1 -> Mux1/3
  Add2/1 -> Mux1/2
  hipM10/1 -> Add2/2
  hipM3/1 -> Add2/1
  Add3/1 -> Mux1/1
  hipM2/1 -> Add3/2
  hipM1/1 -> Add3/1
  Mux1/1 -> [RHSwStim]
  R Swing Phase (sagittal)/8(M10 [HFL GLU VAS]) -> hipM10/1, hipM2/1, "L Stance, Swing, Trans (sagittal)1"/20(S_M10)
  R Swing Phase (sagittal)/7(M9 [HAM BFSH GAS]) -> hipM11/1, "L Stance, Swing, Trans (sagittal)1"/19(S_M9)
  R Swing Phase (sagittal)/6(M8 [RF BFSH]) -> hipM12/1, "L Stance, Swing, Trans (sagittal)1"/18(S_M8)
  R Swing Phase (sagittal)/5(S_M7_Sw [BFSH]) -> "L Stance, Swing, Trans (sagittal)1"/17(S_M7_Sw)
  R Swing Phase (sagittal)/4(S_M7_DS [BFSH]) -> "L Stance, Swing, Trans (sagittal)1"/16(S_M7_DS)
  R Swing Phase (sagittal)/3(S_M6 [HFL GLU]) -> hipM1/1, hipM3/1, "L Stance, Swing, Trans (sagittal)1"/15(S_M6)
  R Swing Phase (sagittal)/2(S_M5_Sw [TA]) -> "L Stance, Swing, Trans (sagittal)1"/14(S_M5_Sw)
  R Swing Phase (sagittal)/1(S_Sw_0) -> "L Stance, Swing, Trans (sagittal)1"/13(S_0_Sw)
  "L Stance, Swing, Trans (sagittal)1"/1(S) -> Saturation1/1
  hipM8/1 -> Mux/4
  hipM9/1 -> Mux/3
  Add1/1 -> Mux/2
  hipM7/1 -> Add1/2
  hipM6/1 -> Add1/1
  Add9/1 -> Mux/1
  hipM5/1 -> Add9/2
  hipM4/1 -> Add9/1
  Mux/1 -> [LHSwStim]
  L Swing Phase (sagittal)/8(M10 [HFL GLU VAS]) -> hipM7/1, hipM5/1, "L Stance, Swing, Trans (sagittal)"/20(S_M10)
  L Swing Phase (sagittal)/7(M9 [HAM BFSH GAS]) -> hipM8/1, "L Stance, Swing, Trans (sagittal)"/19(S_M9)
  L Swing Phase (sagittal)/6(M8 [RF BFSH]) -> hipM9/1, "L Stance, Swing, Trans (sagittal)"/18(S_M8)
  L Swing Phase (sagittal)/5(S_M7_Sw [BFSH]) -> "L Stance, Swing, Trans (sagittal)"/17(S_M7_Sw)
  L Swing Phase (sagittal)/4(S_M7_DS [BFSH]) -> "L Stance, Swing, Trans (sagittal)"/16(S_M7_DS)
  L Swing Phase (sagittal)/3(S_M6 [HFL GLU]) -> hipM4/1, hipM6/1, "L Stance, Swing, Trans (sagittal)"/15(S_M6)
  L Swing Phase (sagittal)/2(S_M5_Sw [TA]) -> "L Stance, Swing, Trans (sagittal)"/14(S_M5_Sw)
  L Stance Phase (sagittal)/5(S_M4 [HFL GLU HAM]) -> "L Stance, Swing, Trans (sagittal)"/11(S_M4)
  L Stance Phase (sagittal)1/5(S_M4 [HFL GLU HAM]) -> "L Stance, Swing, Trans (sagittal)1"/11(S_M4)
  SDelay30/1 -> L Stance Phase (sagittal)1/3(theta dtheta [rad rad/s])
  Mux4/1 -> LL Delay3/1
  LL Delay3/1 -> SDelay30/1
  SDelay29/1 -> L Stance Phase (sagittal)/3(theta dtheta [rad rad/s])
  Mux2/1 -> LL Delay2/1
  LL Delay2/1 -> SDelay29/1
  SDelay3/1 -> "L Stance, Swing, Trans (sagittal)1"/5(ILLoad)
  L Stance Phase (sagittal)1/4(S_M3 [HFL GLU HAM]) -> "L Stance, Swing, Trans (sagittal)1"/10(S_M3)
  L Stance Phase (sagittal)/4(S_M3 [HFL GLU HAM]) -> "L Stance, Swing, Trans (sagittal)"/10(S_M3)
  [theta_tgt] -> L Stance Phase (sagittal)1/2(theta_tgt [rad])
  [dtheta] -> Mux4/2
  [theta] -> Mux4/1
  SDelay/1 -> "L Stance, Swing, Trans (sagittal)"/5(ILLoad)
  [theta_tgt] -> L Stance Phase (sagittal)/2(theta_tgt [rad])
  [dtheta] -> Mux2/2
  [theta] -> Mux2/1
  L Stance Phase (sagittal)1/6(S_M5 [TA]) -> "L Stance, Swing, Trans (sagittal)1"/12(S_M5_St)
  L Stance Phase (sagittal)1/3(S_M2 [HAM VAS BFSH GAS]) -> "L Stance, Swing, Trans (sagittal)1"/9(S_M2)
  L Stance Phase (sagittal)1/2(S_M1 [GLU VAS SOL]) -> "L Stance, Swing, Trans (sagittal)1"/8(S_M1)
  L Stance Phase (sagittal)/6(S_M5 [TA]) -> "L Stance, Swing, Trans (sagittal)"/12(S_M5_St)
  L Stance Phase (sagittal)/3(S_M2 [HAM VAS BFSH GAS]) -> "L Stance, Swing, Trans (sagittal)"/9(S_M2)
  L Stance Phase (sagittal)/2(S_M1 [GLU VAS SOL]) -> "L Stance, Swing, Trans (sagittal)"/8(S_M1)
  L Stance Phase (sagittal)1/1(S_St_0) -> "L Stance, Swing, Trans (sagittal)1"/7(S_0_St)
  L Swing Phase (sagittal)/1(S_Sw_0) -> "L Stance, Swing, Trans (sagittal)"/13(S_0_Sw)
  L Stance Phase (sagittal)/1(S_St_0) -> "L Stance, Swing, Trans (sagittal)"/7(S_0_St)
  SDelay28/1 -> L Swing Phase (sagittal)/3(a_tgt)
  Sum6/1 -> LL Delay1/1
  LL Delay1/1 -> SDelay28/1
  [RLceVAS] -> MDelay15/1
  [RLceGLU] -> SDelay13/1
  [RLceHFL] -> SDelay5/1
  [LLceVAS] -> MDelay5/1
  [LLceGLU] -> SDelay11/1
  [LLceHFL] -> SDelay10/1
  MDelay13/1 -> "L Stance, Swing, Trans (sagittal)1"/3(CStance)
  MDelay14/1 -> "L Stance, Swing, Trans (sagittal)1"/2(Stance)
  MDelay19/1 -> "L Stance, Swing, Trans (sagittal)"/3(CStance)
  MDelay20/1 -> "L Stance, Swing, Trans (sagittal)"/2(Stance)
  [theta] -> Sum1/1
  [Ralpha_tgt] -> Sum1/2
  [theta] -> Sum6/1
  [Lalpha_tgt] -> Sum6/2
  LDelay6/1 -> [RStimTA]
  LDelay8/1 -> [RStimSOL]
  LDelay7/1 -> [RStimGAS]
  MDelay11/1 -> [RStimBFSH]
  MDelay12/1 -> [RStimVAS]
  SDelay27/1 -> [RStimRF]
  SDelay26/1 -> [RStimHAM]
  SDelay25/1 -> [RStimGLU]
  SDelay24/1 -> [RStimHFL]
  Demux4/6 -> MDelay11/1
  Demux4/5 -> MDelay12/1
  Demux4/4 -> SDelay27/1
  Demux4/9 -> LDelay6/1
  Demux4/8 -> LDelay8/1
  Demux4/7 -> LDelay7/1
  Demux4/3 -> SDelay26/1
  Demux4/2 -> SDelay25/1
  Demux4/1 -> SDelay24/1
  LDelay10/1 -> [LStimTA]
  LDelay9/1 -> [LStimSOL]
  LDelay11/1 -> [LStimGAS]
  MDelay10/1 -> [LStimBFSH]
  MDelay9/1 -> [LStimVAS]
  SDelay23/1 -> [LStimRF]
  SDelay22/1 -> [LStimHAM]
  SDelay21/1 -> [LStimGLU]
  SDelay20/1 -> [LStimHFL]
  SDelay12/1 -> "L Stance, Swing, Trans (sagittal)"/6(CLLoad)
  [LStance] -> MDelay13/1
  [RStance] -> MDelay14/1
  [LonR] -> "L Stance, Swing, Trans (sagittal)1"/4(ConI)
  Saturation1/1 -> Demux4/1
  [LLLoad] -> SDelay14/1
  SDelay14/1 -> "L Stance, Swing, Trans (sagittal)1"/6(CLLoad)
  [TrCtrlPar] -> "L Stance, Swing, Trans (sagittal)1"/1(CtrlPar)
  MDelay15/1 -> R Swing Phase (sagittal)/14(LceVAS)
  SDelay13/1 -> R Swing Phase (sagittal)/13(LceGLU)
  SDelay5/1 -> R Swing Phase (sagittal)/12(LceHFL)
  MDelay7/1 -> R Swing Phase (sagittal)/11(VceBFSH)
  [RVceBFSH] -> MDelay7/1
  SDelay19/1 -> R Swing Phase (sagittal)/8(VceHAM)
  [RVceHAM] -> SDelay19/1
  SDelay18/1 -> R Swing Phase (sagittal)/6(VceRF)
  [RVceRF] -> SDelay18/1
  SDelay15/1 -> R Swing Phase (sagittal)/7(LceHAM)
  [RLceHAM] -> SDelay15/1
  SDelay4/1 -> R Swing Phase (sagittal)/5(LceRF)
  [RLceRF] -> SDelay4/1
  [leg_clr] -> R Swing Phase (sagittal)/4(l_clr)
  [LonR] -> Logical Operator2/1
  Logical Operator2/1 -> R Swing Phase (sagittal)/Enable
  Logical Operator1/1 -> Logical Operator2/2
  R Stance afferent delay/1 -> L Stance Phase (sagittal)1/Enable, Logical Operator1/1, R Swing Phase (sagittal)/2(Stance)
  [SwCtrlPar] -> R Swing Phase (sagittal)/1(CtrlPar)
  LDelay5/1 -> L Stance Phase (sagittal)1/11(LceTA), R Swing Phase (sagittal)/15(LceTA)
  [RLceTA] -> LDelay5/1
  LDelay4/1 -> L Stance Phase (sagittal)1/10(FmSOL)
  [RFmSOL] -> LDelay4/1
  LDelay3/1 -> L Stance Phase (sagittal)1/9(FmGAS)
  [RFmGAS] -> LDelay3/1
  MDelay6/1 -> L Stance Phase (sagittal)1/8(LceBFSH), R Swing Phase (sagittal)/9(lceBFSH)
  [RLceBFSH] -> MDelay6/1
  MDelay1/1 -> L Stance Phase (sagittal)1/7(FmVAS)
  [RFmVAS] -> MDelay1/1
  SDelay17/1 -> L Stance Phase (sagittal)1/6(FmHAM)
  [RFmHAM] -> SDelay17/1
  SDelay16/1 -> L Stance Phase (sagittal)1/5(FmGLU)
  [RFmGLU] -> SDelay16/1
  [LHSwStim] -> L Stance Phase (sagittal)1/4(CStim_HSw)
  [RLLoad] -> SDelay3/1
  [StCtrlPar] -> L Stance Phase (sagittal)1/1(CtrlPar)
  Right Stance?1/1 -> Data Type Conversion1/1
  [RStance] -> MDelay19/1
  [LStance] -> MDelay20/1
  [RonL] -> "L Stance, Swing, Trans (sagittal)"/4(ConI)
  "L Stance, Swing, Trans (sagittal)"/1(S) -> Saturation10/1
  Demux3/6 -> MDelay10/1
  Demux3/5 -> MDelay9/1
  Demux3/4 -> SDelay23/1
  Demux3/9 -> LDelay10/1
  Demux3/8 -> LDelay9/1
  Demux3/7 -> LDelay11/1
  Saturation10/1 -> Demux3/1
  Demux3/3 -> SDelay22/1
  Demux3/2 -> SDelay21/1
  Demux3/1 -> SDelay20/1
  [RLLoad] -> SDelay12/1
  [TrCtrlPar] -> "L Stance, Swing, Trans (sagittal)"/1(CtrlPar)
  MDelay5/1 -> L Swing Phase (sagittal)/14(LceVAS)
  SDelay11/1 -> L Swing Phase (sagittal)/13(LceGLU)
  SDelay10/1 -> L Swing Phase (sagittal)/12(LceHFL)
  MDelay4/1 -> L Swing Phase (sagittal)/11(VceBFSH)
  [LVceBFSH] -> MDelay4/1
  SDelay9/1 -> L Swing Phase (sagittal)/8(VceHAM)
  [LVceHAM] -> SDelay9/1
  SDelay8/1 -> L Swing Phase (sagittal)/6(VceRF)
  [LVceRF] -> SDelay8/1
  SDelay2/1 -> L Swing Phase (sagittal)/7(LceHAM)
  [LLceHAM] -> SDelay2/1
  SDelay1/1 -> L Swing Phase (sagittal)/5(LceRF)
  [LLceRF] -> SDelay1/1
  [leg_clr] -> L Swing Phase (sagittal)/4(l_clr)
  [RonL] -> Logical Operator3/1
  Logical Operator3/1 -> L Swing Phase (sagittal)/Enable
  Logical Operator/1 -> Logical Operator3/2
  L Stance afferent delay/1 -> L Swing Phase (sagittal)/2(Stance), Logical Operator/1, L Stance Phase (sagittal)/Enable
  [SwCtrlPar] -> L Swing Phase (sagittal)/1(CtrlPar)
  LDelay2/1 -> L Stance Phase (sagittal)/11(LceTA), L Swing Phase (sagittal)/15(LceTA)
  [LLceTA] -> LDelay2/1
  LDelay1/1 -> L Stance Phase (sagittal)/10(FmSOL)
  [LFmSOL] -> LDelay1/1
  LDelay/1 -> L Stance Phase (sagittal)/9(FmGAS)
  [LFmGAS] -> LDelay/1
  MDelay3/1 -> L Stance Phase (sagittal)/8(LceBFSH), L Swing Phase (sagittal)/9(lceBFSH)
  [LLceBFSH] -> MDelay3/1
  MDelay2/1 -> L Stance Phase (sagittal)/7(FmVAS)
  [LFmVAS] -> MDelay2/1
  SDelay7/1 -> L Stance Phase (sagittal)/6(FmHAM)
  [LFmHAM] -> SDelay7/1
  SDelay6/1 -> L Stance Phase (sagittal)/5(FmGLU)
  [LFmGLU] -> SDelay6/1
  [RHSwStim] -> L Stance Phase (sagittal)/4(CStim_HSw)
  [StCtrlPar] -> L Stance Phase (sagittal)/1(CtrlPar)
  Left Stance?2/1 -> Data Type Conversion/1
  [LLLoad] -> SDelay/1
  9/1 -> Left Stance?2/1
  8/1 -> Left Stance?2/2
  7/1 -> Left Stance?2/3
  " 2"/1 -> Left Stance?2/4
  [phase] -> " 2"/1, 7/1, 9/1, 8/1
  12/1 -> Right Stance?1/1
  11/1 -> Right Stance?1/2
  10/1 -> Right Stance?1/3
  " 3"/1 -> Right Stance?1/4
  [phase] -> " 3"/1, 10/1, 12/1, 11/1
  Data Type Conversion/1 -> [LStance], L Stance afferent delay/1
  Data Type Conversion1/1 -> [RStance], R Stance afferent delay/1

== system nmc/NMC Model/etc ==
  note: Control Parameters
  Clock : Clock
  Constant{1,7,13..18,20,22} (10 alike) : Constant  Value=CtrlPar_VelocityFile_List
  Constant10 : Constant  Value=CtrlPar_Tr_List
  Constant11 : Constant  Value=CtrlPar_Tr_R_List
  Constant12 : Constant  Value=CtrlPar_theta0_List
  Constant2 : Constant  Value=CtrlPar_LL_List
  Constant3 : Constant  Value=CtrlPar_St_R_List
  Constant4 : Constant  Value=CtrlPar_FP_R_List
  Constant5 : Constant  Value=CtrlPar_St_List
  Constant6 : Constant  Value=CtrlPar_FP_List
  Constant8 : Constant  Value=CtrlPar_Sw_R_List
  Constant9 : Constant  Value=CtrlPar_Sw_List
  ParamScaling{,1..9} (10 alike) : nmc/ParamScaling
  To Current Workspace2 : ToWorkspace  VariableName=simout_tEnd  SaveFormat=Structure  SampleTime=-1
      settings: MaxDataPoints=1
  tag scope: FPCtrlPar=global, LLCtrlPar=global, R_FPCtrlPar=global, R_StCtrlPar=global, R_SwCtrlPar=global, R_TrCtrlPar=global, StCtrlPar=global, SwCtrlPar=global, TrCtrlPar=global, theta0=global
  wires:
  Clock/1 -> To Current Workspace2/1
  Constant4/1 -> ParamScaling/1
  ParamScaling/1 -> [R_FPCtrlPar]
  [NMC_CurVelocity] -> ParamScaling/3
  Constant13/1 -> ParamScaling/2
  Constant8/1 -> ParamScaling1/1
  ParamScaling1/1 -> [R_SwCtrlPar]
  [NMC_CurVelocity] -> ParamScaling1/3
  Constant1/1 -> ParamScaling1/2
  Constant11/1 -> ParamScaling2/1
  ParamScaling2/1 -> [R_TrCtrlPar]
  [NMC_CurVelocity] -> ParamScaling2/3
  Constant14/1 -> ParamScaling2/2
  Constant12/1 -> ParamScaling3/1
  ParamScaling3/1 -> [theta0]
  [NMC_CurVelocity] -> ParamScaling3/3
  Constant16/1 -> ParamScaling3/2
  Constant6/1 -> ParamScaling4/1
  ParamScaling4/1 -> [FPCtrlPar]
  [NMC_CurVelocity] -> ParamScaling4/3
  Constant18/1 -> ParamScaling4/2
  Constant2/1 -> ParamScaling5/1
  ParamScaling5/1 -> [LLCtrlPar]
  [NMC_CurVelocity] -> ParamScaling5/3
  Constant20/1 -> ParamScaling5/2
  Constant5/1 -> ParamScaling6/1
  ParamScaling6/1 -> [StCtrlPar]
  [NMC_CurVelocity] -> ParamScaling6/3
  Constant22/1 -> ParamScaling6/2
  Constant9/1 -> ParamScaling7/1
  ParamScaling7/1 -> [SwCtrlPar]
  [NMC_CurVelocity] -> ParamScaling7/3
  Constant7/1 -> ParamScaling7/2
  Constant10/1 -> ParamScaling8/1
  ParamScaling8/1 -> [TrCtrlPar]
  [NMC_CurVelocity] -> ParamScaling8/3
  Constant15/1 -> ParamScaling8/2
  Constant3/1 -> ParamScaling9/1
  ParamScaling9/1 -> [R_StCtrlPar]
  [NMC_CurVelocity] -> ParamScaling9/3
  Constant17/1 -> ParamScaling9/2

== system nmc/NMC Model/Global to Body frame/body pitch//roll//yaw in body frame --- x-axis: forward y-axis: leftward z-axis: parallel to gravity ==
  LHip : Inport
  dLHip : Inport  Port=2
  HAT : Inport  Port=3
  dHAT : Inport  Port=4
  RHip : Inport  Port=5
  dRHip : Inport  Port=6
  " Mean Hip Speed" : Gain  Gain=1/2
  "Dx, Dy" : Selector  InputPortWidth=3  IndexOptions=Index vector (dialog)  Indices=[1 2]  OutputSizes=1
  "Dx, Dz" : Selector  InputPortWidth=3  IndexOptions=Index vector (dialog)  Indices=[1 3]  OutputSizes=1
  "Dx, Dz1" : Selector  InputPortWidth=3  IndexOptions=Index vector (dialog)  Indices=[1 3]  OutputSizes=1
  "Dz, Dy" : Selector  InputPortWidth=3  IndexOptions=Index vector (dialog)  Indices=[3 2]  OutputSizes=1
  Mean Hip Position : Gain  Gain=1/2
  Mux1 : Mux  Inputs=2
  Mux2 : Mux  Inputs=2
  Mux3 : Mux  Inputs=2
  Sum1 : Sum
  Sum2 : Sum
  Sum4 : Sum  Inputs=-+
  Sum5 : Sum  Inputs=+-
  Theta : Fcn  Expr=atan2(u(1),u(2))
  Theta1 : Fcn  Expr=atan2(u(1),u(2))
  "dDx, dDy" : Selector  InputPortWidth=3  IndexOptions=Index vector (dialog)  Indices=[1 2]  OutputSizes=1
  "dDz, dDy" : Selector  InputPortWidth=3  IndexOptions=Index vector (dialog)  Indices=[3 2]  OutputSizes=1
  dTheta : Fcn  Expr=( u(2)*u(3) - u(1)*u(4) ) / D1G_HAT^2
  dTheta1 : Fcn  Expr=( u(2)*u(3) - u(1)*u(4) ) / D1G_HAT^2
  map1 : Subsystem
  map2 : Subsystem
  new_bases : Subsystem
  yaw1 : Fcn  Expr=atan2(-u(1)+u(3),-u(2)+u(4))
  th_pitch : Outport
  dth_pitch : Outport  Port=2
  th_roll : Outport  Port=3
  dth_roll : Outport  Port=4
  yaw : Outport  Port=5
  wires:
  dHAT/1 -> Sum5/1
  "dDx, dDy"/1 -> Mux2/2
  Mux2/1 -> dTheta/1
  Sum1/1 -> Mean Hip Position/1
  Sum2/1 -> " Mean Hip Speed"/1
  HAT/1 -> Sum4/2
  Mean Hip Position/1 -> Sum4/1
  " Mean Hip Speed"/1 -> Sum5/2
  "Dx, Dy"/1 -> Mux2/1, Theta/1
  LHip/1 -> Sum1/1, new_bases/1(L), "Dx, Dz"/1
  RHip/1 -> Sum1/2, new_bases/2(R), "Dx, Dz1"/1
  dLHip/1 -> Sum2/1
  dRHip/1 -> Sum2/2
  Theta/1 -> th_pitch/1
  dTheta/1 -> dth_pitch/1
  Sum4/1 -> map1/1(v)
  map1/1(v_new) -> "Dx, Dy"/1, "Dz, Dy"/1
  new_bases/1(bases) -> map1/2(basis), map2/2(basis)
  Sum5/1 -> map2/1(v)
  map2/1(v_new) -> "dDx, dDy"/1, "dDz, dDy"/1
  "dDz, dDy"/1 -> Mux1/2
  Mux1/1 -> dTheta1/1
  "Dz, Dy"/1 -> Mux1/1, Theta1/1
  Theta1/1 -> th_roll/1
  dTheta1/1 -> dth_roll/1
  "Dx, Dz"/1 -> Mux3/1
  "Dx, Dz1"/1 -> Mux3/2
  Mux3/1 -> yaw1/1
  yaw1/1 -> yaw/1
